simulink model "NeuroMuscular"  (Simulink 6.4)
settings: Solver=ode45  StartTime=0.0  StopTime=10.0  RelTol=1e-3
values from neighbouring files (symbols this model uses):
  DtotalIC = 0.3    [NeuroMuscular_IC.m]    (also in Respiratory_IC.m = 0.32)
  Mueller_activation = 0    [NeuroMuscular_IC.m]
  t_Mueller_duration = 0    [NeuroMuscular_IC.m]
  t_Mueller_insp = 0    [NeuroMuscular_IC.m]
  t_Mueller_start = 0    [NeuroMuscular_IC.m]
  t_valsalva_duration = 0    [NeuroMuscular_IC.m]
  t_valsalva_insp = 0    [NeuroMuscular_IC.m]
  t_valsalva_start = 0    [NeuroMuscular_IC.m]
  Td = Td_new    [acquire_data.m]    (also in acquire_data_save.m)
  time_step = time_step    [acquire_data.m]    (also in acquire_data_save.m)
  TImean = 1.5    [NeuroMuscular_IC.m]    (also in Respiratory_IC.m)
  TTmean = 4.0    (= 4)    [NeuroMuscular_IC.m]    (also in Respiratory_IC.m)
  Valsalva_activation = 0    [NeuroMuscular_IC.m]
undefined symbols (not defined in the file or in its folder): first_time, resp_period_end
settings Model: LastModifiedBy=CLM
settings OptimizationCC: BlockReduction=off  BooleanDataType=off
settings DebuggingCC: SolverPrmCheckMsg=none  StrictBusMsg=None
settings HardwareCC: TargetUnknown=on

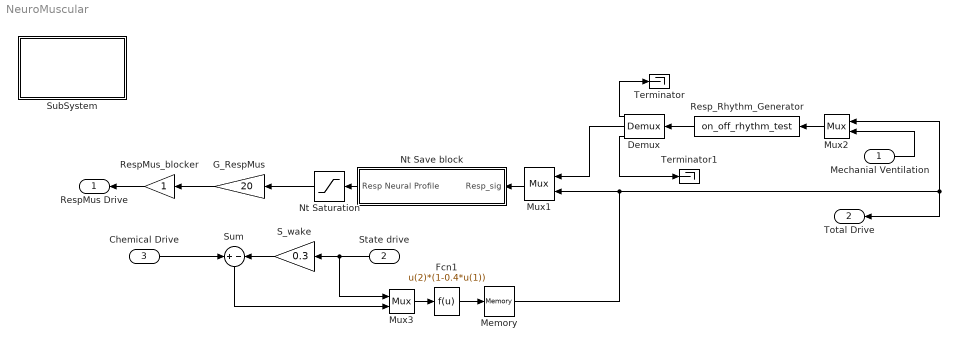
== system NeuroMuscular ==
  Mechanial Ventilation : Inport
  State drive : Inport  Orientation=left  Port=2
  Chemical Drive : Inport  Port=3
  Demux : Demux  Orientation=left  Outputs=3
  Fcn1 : Fcn  Expr=u(2)*(1-0.4*u(1))
  G_RespMus : Gain  Orientation=left  Gain=20  SaturateOnIntegerOverflow=on
  Memory : Memory  X0=DtotalIC
  Mux1 : Mux  Orientation=left  Inputs=2
  Mux2 : Mux  Orientation=left  Inputs=2
  Mux3 : Mux  Inputs=2
  Nt Saturation : Saturate  Orientation=left  UpperLimit=10  LowerLimit=0
  Nt Save block : Subsystem  Orientation=left
  RespMus_blocker : Gain  Orientation=left  SaturateOnIntegerOverflow=on
  Resp_Rhythm_Generator : S-Function  Orientation=left  FunctionName=on_off_rhythm_test  Parameters=t_valsalva_start,t_valsalva_duration,Valsalva_activation,t_valsalva_insp,t_Mueller_start,t_Mueller_duration,Mueller_activation,t_Mueller_insp,TTmean,TImean,Td,first_time,resp_period_end,time_step
  S_wake : Gain  Orientation=left  Gain=0.3  SaturateOnIntegerOverflow=on
  SubSystem : Subsystem
      settings: OpenFcn=NeuroMuscular_IC
      mask Display: disp('"double click here"\n to load \nNeuroMuscular \ninitial values');
  Sum : Sum  Orientation=down  Inputs=+-  SaturateOnIntegerOverflow=on  InputSameDT=on
  Terminator : Terminator
  Terminator1 : Terminator
  "RespMus Drive " : Outport  Orientation=left
  Total Drive : Outport  Orientation=left  Port=2
  wires:
  Memory/1 -> Total Drive/1, Mux2/1, Mux1/2
  Mechanial Ventilation/1 -> Mux2/2
  Mux2/1 -> Resp_Rhythm_Generator/1
  Demux/1 -> Terminator/1
  Demux/3 -> Terminator1/1
  Nt Save block/1(Resp Neural Profile) -> Nt Saturation/1
  Sum/1 -> Mux3/2
  Fcn1/1 -> Memory/1
  Mux3/1 -> Fcn1/1
  Demux/2 -> Mux1/1
  Nt Saturation/1 -> G_RespMus/1
  Chemical Drive/1 -> Sum/1
  State drive/1 -> S_wake/1, Mux3/1
  Mux1/1 -> Nt Save block/1(Resp_sig)
  Resp_Rhythm_Generator/1 -> Demux/1
  S_wake/1 -> Sum/2
  G_RespMus/1 -> RespMus_blocker/1
  RespMus_blocker/1 -> "RespMus Drive "/1

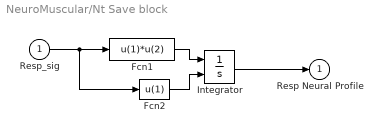
== system NeuroMuscular/Nt Save block ==
  Resp_sig : Inport
  Fcn1 : Fcn  Expr=u(1)*u(2)
  Fcn2 : Fcn  Expr=u(1)
  Integrator : Integrator  ExternalReset=falling
  Resp Neural Profile : Outport
  wires:
  Fcn2/1 -> Integrator/2
  Fcn1/1 -> Integrator/1
  Resp_sig/1 -> Fcn2/1, Fcn1/1
  Integrator/1 -> Resp Neural Profile/1

== system NeuroMuscular/SubSystem ==
